simulink model "commadjcochanint1"  (R2018b)
settings: Solver=VariableStepDiscrete  StartTime=0.0  StopTime=0.1  RelTol=1e-3  AbsTol=1e-6
libraries: commdigbbndpm3 x4, commfilt2 x4, commrandsrc3 x3, simulink x2, dspmathops x2, commrflib2 x2, commchan3 x1, commsink2 x1, commblksprivate x1
Description:
  | Adjacent and Co-Channel Interference
settings Model: RequirementInfo=9  ExtModeTrigMode=oneshot  ExtModeArmWhenConnect=off  ExtModeAutoUpdateStatusClock=off  Creator=The MathWorks, Inc.  LastModifiedBy=Aviya
settings SolverCC: AutoScaleAbsTol=off  InsertRTBMode=Auto
settings DataIOCC: SaveFormat=Array  SaveOutput=off  SaveTime=off  SignalLoggingName=adjcoSigsOut
settings OptimizationCC: BlockReduction=off  BooleanDataType=off  ExpressionDepthLimit=2147483647  InitFltsAndDblsToZero=on  EfficientMapNaN2IntZero=off  LifeSpan=inf
settings DebuggingCC: UnderspecifiedInitializationDetection=Classic  MergeDetectMultiDrivingBlocksExec=none  CheckExecutionContextPreStartOutputMsg=on  CheckExecutionContextRuntimeOutputMsg=on  SignalResolutionControl=TryResolveAllWithWarning  InheritedTsInSrcMsg=none  MultiTaskDSMMsg=warning  MultiTaskCondExecSysMsg=none  SigSpecEnsureSampleTimeMsg=none  IntegerOverflowMsg=none  FcnCallInpInsideContextMsg=warning  AllowSymbolicDim=off  StateNameClashWarn=warning  SFUnexpectedBacktrackingDiag=warning  SFNoUnconditionalDefaultTransitionDiag=warning  SFExecutionAtInitializationDiag=none  IntegerSaturationMsg=none
settings HardwareCC: ProdBitPerPointer=32  ProdBitPerSizeT=32  ProdBitPerPtrDiffT=32  ProdLargestAtomicFloat=None  ProdIntDivRoundTo=Undefined  ProdEndianess=Unspecified  ProdWordSize=32  ProdHWDeviceType=Specified
settings ModelReferenceCC: UpdateModelReferenceTargets=IfOutOfDate  PropagateSignalLabelsOutOfModel=off
settings SFSimCC: SimUseLocalCustomCode=off
settings RTWCC: RTWUseLocalCustomCode=off
settings CodeAppCC: MangleLength=5  StateflowObjectComments=on
settings GRTTargetCC: TargetFcnLib=ansi_tfl_tmw_new.mat  TargetLangStandard=C89/C90 (ANSI)  GeneratePreprocessorConditionals=Disable all  CombineOutputUpdateFcns=off  GRTInterface=on
settings ConfigComp: CovMetricSettings=d  CovHtmlReporting=on  CovSaveCumulativeToWorkspaceVar=on  CovSaveSingleToWorkspaceVar=on  CovExternalEMLEnable=off  CovSFcnEnable=off

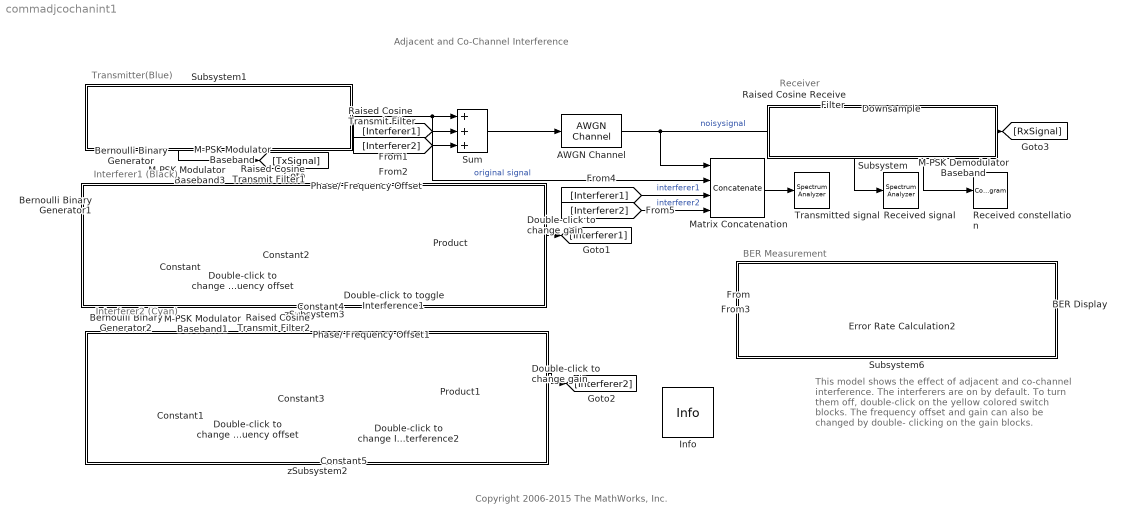
== system commadjcochanint1 ==
  note: Adjacent and Co-Channel Interference
  note: Interferer1 (Black)
  note: Transmitter(Blue)
  note: Interferer2 (Cyan)
  note: Receiver
  note: BER Measurement
  note: This model shows the effect of adjacent
      | and co-channel interference. The interferers are
      | on by default. To turn them off, double-click on
      | the yellow colored switch blocks. The frequency
      | offset and gain can also be changed by double-
      | clicking on the gain blocks.
  note: Copyright 2006-2015 The MathWorks, Inc.
  AWGN Channel : commchan3/AWGN Channel  InputProcessing=Columns as channels (frame based)  seed=123456  noiseMode="Signal to noise ratio  (Es/No)"  EbNodB=10  EsNodB=30  SNRdB=10  bitsPerSym=1  Ps=1/8  Tsym=1e-6  variance=1
  BER Display : Display
  Bernoulli Binary Generator : commrandsrc3/Bernoulli Binary Generator  ProbabilityOfZero=0.5  SeedSource=Parameter  Seed=529558  SampleTime=1e-6/3  SamplesPerFrame=300  OutputDataType=boolean  SimulateUsing=Interpreted execution
  Bernoulli Binary Generator1 : commrandsrc3/Bernoulli Binary Generator  ProbabilityOfZero=0.5  SeedSource=Parameter  Seed=529573  SampleTime=1e-6/3  SamplesPerFrame=300  OutputDataType=boolean  SimulateUsing=Interpreted execution
  Bernoulli Binary Generator2 : commrandsrc3/Bernoulli Binary Generator  ProbabilityOfZero=0.5  SeedSource=Parameter  Seed=529397  SampleTime=1e-6/3  SamplesPerFrame=300  OutputDataType=boolean  SimulateUsing=Interpreted execution
  Constant : Constant  Value=-4e6  VectorParams1D=off  SampleTime=(1e-6/3)*300
  Constant1 : Constant  Value=4e6  VectorParams1D=off  SampleTime=(1e-6/3)*300
  Constant2 : Constant  Value=0  VectorParams1D=off  SampleTime=(1e-6/3)*300
  Constant3 : Constant  Value=0  VectorParams1D=off  SampleTime=(1e-6/3)*300
  Constant4 : Constant  VectorParams1D=off  SampleTime=(1e-6/3)*300
  Constant5 : Constant  VectorParams1D=off  SampleTime=(1e-6/3)*300
  Double-click to change Interference2 : ManualSwitch  CurrentSetting=0
  Double-click to change frequency offset : simulink/Math Operations/Slider Gain  gain=0.5  low=-0.85  high=0.85
  Double-click to change gain : dspmathops/dB Gain  dB=-20  intype=Amplitude
      settings: SourceProductName=DSP System Toolbox  SourceProductBaseCode=DS
  "Double-click to change gain " : dspmathops/dB Gain  dB=-10  intype=Amplitude
      settings: SourceProductName=DSP System Toolbox  SourceProductBaseCode=DS
  Double-click to toggle Interference1 : ManualSwitch  CurrentSetting=0
  Double-click to change frequency offset : simulink/Math Operations/Slider Gain  gain=0.5  low=-0.85  high=0.85
  Downsample : DownSample  N=8
  Error Rate Calculation2 : commsink2/Error Rate Calculation  N=12*3  st_delay=0  cp_mode=Entire frame  subframe=[]  PMode=Port  WsName=e1  RsMode2=off  stop=off  numErr=100  maxBits=1e6
  Info : commblksprivate/Info  SystemSampleTime=-1
      settings: SourceProductName=Communications System Toolbox  SourceProductBaseCode=CM
  M-PSK Demodulator Baseband : commdigbbndpm3/M-PSK Demodulator Baseband  M=8  OutType=Bit  DecType=Hard decision  VarSource=Dialog  Variance=1  Dec=Gray  Mapping=[0:7]  Ph=0  outDtype1=boolean  outDtype2=double  derotateFactorWordLen=16  derotateFactorDataTypeStr=Inherit: Same word length as input  derotateFactorLastDataTypeStr=Inherit: Same word length as input
      settings: SourceProductName=Communications System Toolbox
  M-PSK Modulator Baseband : commdigbbndpm3/M-PSK Modulator Baseband  M=8  InType=Bit  Enc=Gray  Mapping=0  Ph=0  outDtype=double  outWordLen=16  outUDDataType=sfix(16)  outFracLenMode=Best precision  outFracLen=15  outDataTypeStr=double  outLastDataTypeStr=double
      settings: SourceProductName=Communications System Toolbox
  M-PSK Modulator Baseband1 : commdigbbndpm3/M-PSK Modulator Baseband  M=8  InType=Bit  Enc=Gray  Mapping=0  Ph=0  outDtype=double  outWordLen=16  outUDDataType=sfix(16)  outFracLenMode=Best precision  outFracLen=15  outDataTypeStr=double  outLastDataTypeStr=double
      settings: SourceProductName=Communications System Toolbox
  M-PSK Modulator Baseband3 : commdigbbndpm3/M-PSK Modulator Baseband  M=8  InType=Bit  Enc=Gray  Mapping=0  Ph=0  outDtype=double  outWordLen=16  outUDDataType=sfix(16)  outFracLenMode=Best precision  outFracLen=15  outDataTypeStr=double  outLastDataTypeStr=double
      settings: SourceProductName=Communications System Toolbox
  Matrix Concatenation : Concatenate  NumInputs=4  Mode=Multidimensional array  ConcatenateDimension=2
  Phase/ Frequency Offset : commrflib2/Phase// Frequency Offset  phaseOffset=0  freqPort=on  freqOffset=0
      settings: SourceProductName=Communications System Toolbox
  Phase/ Frequency Offset1 : commrflib2/Phase// Frequency Offset  phaseOffset=0  freqPort=on  freqOffset=0
      settings: SourceProductName=Communications System Toolbox
  Product : Product  SaturateOnIntegerOverflow=on  OutDataTypeStr=Inherit: Same as first input
  Product1 : Product  SaturateOnIntegerOverflow=on  OutDataTypeStr=Inherit: Same as first input
  Raised Cosine Receive Filter : commfilt2/Raised Cosine Receive Filter  filtType=Square root  R=0.22  filtSpan=12  N=8  downFactor=1  downOffset=0  filterGain=1  InputProcessing=Columns as channels (frame based)  RateOptions=Enforce single-rate processing  framing=Mute  checkCoeff=off  variableName=rcRxFilt  currentFiltSpan=12  D=6  inputOffset=0  sampMode=Mute  saveAsFlag=0  rateMode=Downsampling  checkGain=Normalized  launchFVT=off  roundingMode=Floor  overflowMode=off  coeffDataTypeStr=Inherit: Same word length as input  coeffMin=[]  coeffMax=[]  coeffLastDataTypeStr=Inherit: Same word length as input  accumDataTypeStr=Inherit: Same as product output  accumLastDataTypeStr=Inherit: Same as product output  outputDataTypeStr=Inherit: Same as accumulator  outputMin=[]  outputMax=[]  outputLastDataTypeStr=Inherit: Same as accumulator
  Raised Cosine Transmit Filter : commfilt2/Raised Cosine Transmit Filter  filtType=Square root  R=0.22  filtSpan=12  N=8  filterGain=1  InputProcessing=Columns as channels (frame based)  RateOptions=Enforce single-rate processing  framing=Mute  checkCoeff=off  variableName=rcTxFilt  checkGain=Normalized  sampMode=Mute  saveAsFlag=0  currentFiltSpan=12  D=6  launchFVT=off  roundingMode=Floor  overflowMode=off  coeffDataTypeStr=Inherit: Same word length as input  coeffMin=[]  coeffMax=[]  coeffLastDataTypeStr=Inherit: Same word length as input  outputDataTypeStr=Inherit: Same as accumulator  outputMin=[]  outputMax=[]  outputLastDataTypeStr=Inherit: Same as accumulator
  Raised Cosine Transmit Filter1 : commfilt2/Raised Cosine Transmit Filter  filtType=Square root  R=0.22  filtSpan=12  N=8  filterGain=1  InputProcessing=Columns as channels (frame based)  RateOptions=Enforce single-rate processing  framing=Mute  checkCoeff=off  variableName=rcTxFilt1  checkGain=Normalized  sampMode=Mute  saveAsFlag=0  currentFiltSpan=12  D=6  launchFVT=off  roundingMode=Floor  overflowMode=off  coeffDataTypeStr=Inherit: Same word length as input  coeffMin=[]  coeffMax=[]  coeffLastDataTypeStr=Inherit: Same word length as input  outputDataTypeStr=Inherit: Same as accumulator  outputMin=[]  outputMax=[]  outputLastDataTypeStr=Inherit: Same as accumulator
  Raised Cosine Transmit Filter2 : commfilt2/Raised Cosine Transmit Filter  filtType=Square root  R=0.22  filtSpan=12  N=8  filterGain=1  InputProcessing=Columns as channels (frame based)  RateOptions=Enforce single-rate processing  framing=Mute  checkCoeff=off  variableName=rcTxFilt2  checkGain=Normalized  sampMode=Mute  saveAsFlag=0  currentFiltSpan=12  D=6  launchFVT=off  roundingMode=Floor  overflowMode=off  coeffDataTypeStr=Inherit: Same word length as input  coeffMin=[]  coeffMax=[]  coeffLastDataTypeStr=Inherit: Same word length as input  outputDataTypeStr=Inherit: Same as accumulator  outputMin=[]  outputMax=[]  outputLastDataTypeStr=Inherit: Same as accumulator
  Received constellation : ConstellationDiagram  Tag=ScatterPlot
  Received signal : SpectrumAnalyzer
  Subsystem : Subsystem
      mask Display: disp('');
  Subsystem1 : Subsystem
      mask Display: disp('');
  Subsystem6 : Subsystem
      mask Display: disp('');
  Sum : Sum  Inputs=+++  SaturateOnIntegerOverflow=on
  Transmitted signal : SpectrumAnalyzer
  zSubsystem2 : Subsystem
      mask Display: disp('');
  zSubsystem3 : Subsystem
      mask Display: disp('');
  wires:
  M-PSK Modulator Baseband/1 -> Raised Cosine Transmit Filter/1
  M-PSK Modulator Baseband1/1 -> Raised Cosine Transmit Filter2/1
  M-PSK Modulator Baseband3/1 -> Raised Cosine Transmit Filter1/1
  Raised Cosine Transmit Filter1/1 -> Phase/ Frequency Offset/1
  Raised Cosine Transmit Filter2/1 -> Phase/ Frequency Offset1/1
  Raised Cosine Transmit Filter/1 -> Sum/1, Matrix Concatenation/2  "original signal"
  Constant2/1 -> Double-click to toggle Interference1/1
  Double-click to toggle Interference1/1 -> Product/2
  Constant4/1 -> Double-click to toggle Interference1/2
  Constant3/1 -> Double-click to change Interference2/1
  Double-click to change Interference2/1 -> Product1/2
  Constant5/1 -> Double-click to change Interference2/2
  Phase/ Frequency Offset1/1 -> Product1/1
  Double-click to change frequency offset/1 -> Phase/ Frequency Offset/2
  Constant/1 -> Double-click to change frequency offset/1
  Constant1/1 -> Double-click to change frequency offset/1
  Double-click to change frequency offset/1 -> Phase/ Frequency Offset1/2
  Phase/ Frequency Offset/1 -> Product/1
  Sum/1 -> AWGN Channel/1
  AWGN Channel/1 -> Raised Cosine Receive Filter/1, Matrix Concatenation/1  "noisysignal"
  Raised Cosine Receive Filter/1 -> Received signal/1, Downsample/1
  Downsample/1 -> Received constellation/1, M-PSK Demodulator Baseband/1
  M-PSK Demodulator Baseband/1 -> [RxSignal]
  Product/1 -> Double-click to change gain/1
  Product1/1 -> "Double-click to change gain "/1
  [Interferer1] -> Sum/2
  [Interferer2] -> Sum/3
  Matrix Concatenation/1 -> Transmitted signal/1
  [TxSignal] -> Error Rate Calculation2/1
  [RxSignal] -> Error Rate Calculation2/2
  Double-click to change gain/1 -> [Interferer1]
  "Double-click to change gain "/1 -> [Interferer2]
  [Interferer1] -> Matrix Concatenation/3  "interferer1"
  [Interferer2] -> Matrix Concatenation/4  "interferer2"
  Error Rate Calculation2/1 -> BER Display/1
  Bernoulli Binary Generator/1 -> M-PSK Modulator Baseband/1, [TxSignal]
  Bernoulli Binary Generator1/1 -> M-PSK Modulator Baseband3/1
  Bernoulli Binary Generator2/1 -> M-PSK Modulator Baseband1/1

== system commadjcochanint1/Subsystem ==

== system commadjcochanint1/Subsystem1 ==

== system commadjcochanint1/Subsystem6 ==

== system commadjcochanint1/zSubsystem2 ==

== system commadjcochanint1/zSubsystem3 ==
